simulink library "mylib"  (R2020a)
settings: Solver=VariableStepAuto  StartTime=0.0  StopTime=10.0  RelTol=1e-3
undefined symbols (not defined in the file): d_du_max_pu, dir_to_bus1, dir_to_bus_0L, dir_to_bus_2, dir_to_line1, dir_to_line_0L, dir_to_line_2, du_max_pu, du_ph_max_pu, Fi_0, Fi_T_H, Fi_T_L, Fi_T_M, I0_calc_0L, I0_comp_H, I0_comp_L, I0_comp_M, I0_max_0L, I2_max_2, I_diff1, I_diff2, I_diff3, I_diff4, I_diff5, I_diff_to, I_hight_CT1_G, I_hight_CT2_G, I_low_CT1, I_low_CT2, I_max1, I_max2, I_max3, I_max4, I_max5, I_min_sec_CT1, I_min_sec_CT2, I_unb, Iph_max_0L, Iph_max_2, jmp_in_zone, jmp_in_zone_0L, jmp_in_zone_2, K_dop, max_min1, only_K1_0L, only_K1_2, only_K2_0L, only_K2_2, only_K3_0L, only_K3_2, P_ctl_0, PQ_Fi_ctl_0, Q_ctl_0, S_set_0, set, set1, T_fast, T_I_ctl, T_off, T_on ... (+15)
libraries: $bdroot x184, powerlib_meascontrol x97
(part 14 of 14)

== system mylib/278_dzt_v1/diff_brake/calc_brake_Ic/cut_brake_4/z_ch ==
  in1 : Inport
  in2 : Inport  Port=2
  1 : RelationalOperator  Operator===  OutDataTypeStr=boolean  RndMeth=Simplest
  2 : RelationalOperator  Operator===  OutDataTypeStr=boolean  RndMeth=Simplest
  3 : Logic  AllPortsSameDT=off  OutDataTypeStr=boolean
  36 : Constant  Value=0
  out : Outport
  wires:
  3/1 -> out/1
  2/1 -> 3/2
  1/1 -> 3/1
  36/1 -> 2/2, 1/2
  in2/1 -> 2/1
  in1/1 -> 1/1

== system mylib/278_dzt_v1/diff_brake/calc_brake_Ic/cut_brake_4/z_ch1 ==
  in1 : Inport
  in2 : Inport  Port=2
  1 : RelationalOperator  Operator===  OutDataTypeStr=boolean  RndMeth=Simplest
  2 : RelationalOperator  Operator===  OutDataTypeStr=boolean  RndMeth=Simplest
  3 : Logic  AllPortsSameDT=off  OutDataTypeStr=boolean
  36 : Constant  Value=0
  out : Outport
  wires:
  3/1 -> out/1
  2/1 -> 3/2
  1/1 -> 3/1
  36/1 -> 2/2, 1/2
  in2/1 -> 2/1
  in1/1 -> 1/1

== system mylib/278_dzt_v1/diff_brake/calc_brake_Ic/cut_brake_4/z_ch2 ==
  in1 : Inport
  in2 : Inport  Port=2
  1 : RelationalOperator  Operator===  OutDataTypeStr=boolean  RndMeth=Simplest
  2 : RelationalOperator  Operator===  OutDataTypeStr=boolean  RndMeth=Simplest
  3 : Logic  AllPortsSameDT=off  OutDataTypeStr=boolean
  36 : Constant  Value=0
  out : Outport
  wires:
  3/1 -> out/1
  2/1 -> 3/2
  1/1 -> 3/1
  36/1 -> 2/2, 1/2
  in2/1 -> 2/1
  in1/1 -> 1/1

== system mylib/st_inverse/Inverse time-delay/ANSI Inverse time-delay/Equation ANSI/Zero_check ==
  in : Inport
  Constant : Constant  Value=0
  Constant1 : Constant  Value=0.000001
  Relational Operator : RelationalOperator  Operator===  OutDataTypeStr=boolean  RndMeth=Simplest
  Switch : Switch  Criteria=u2 > Threshold
  out : Outport
  wires:
  in/1 -> Switch/3, Relational Operator/1
  Constant/1 -> Relational Operator/2
  Relational Operator/1 -> Switch/2
  Constant1/1 -> Switch/1
  Switch/1 -> out/1

== system mylib/st_inverse/Inverse time-delay/ANSI Inverse time-delay/Equation ANSI/Zero_check1 ==
  in : Inport
  Constant : Constant  Value=0
  Constant1 : Constant  Value=0.000001
  Relational Operator : RelationalOperator  Operator===  OutDataTypeStr=boolean  RndMeth=Simplest
  Switch : Switch  Criteria=u2 > Threshold
  out : Outport
  wires:
  in/1 -> Switch/3, Relational Operator/1
  Constant/1 -> Relational Operator/2
  Relational Operator/1 -> Switch/2
  Constant1/1 -> Switch/1
  Switch/1 -> out/1

== system mylib/st_inverse/Inverse time-delay/ANSI Inverse time-delay inductive disk relay/Equation ANSI_idr/Zero_check ==
  in : Inport
  Constant : Constant  Value=0
  Constant1 : Constant  Value=0.000001
  Relational Operator : RelationalOperator  Operator===  OutDataTypeStr=boolean  RndMeth=Simplest
  Switch : Switch  Criteria=u2 > Threshold
  out : Outport
  wires:
  in/1 -> Switch/3, Relational Operator/1
  Constant/1 -> Relational Operator/2
  Relational Operator/1 -> Switch/2
  Constant1/1 -> Switch/1
  Switch/1 -> out/1

== system mylib/st_inverse/Inverse time-delay/ANSI Inverse time-delay inductive disk relay/Equation ANSI_idr/Zero_check1 ==
  in : Inport
  Constant : Constant  Value=0
  Constant1 : Constant  Value=0.000001
  Relational Operator : RelationalOperator  Operator===  OutDataTypeStr=boolean  RndMeth=Simplest
  Switch : Switch  Criteria=u2 > Threshold
  out : Outport
  wires:
  in/1 -> Switch/3, Relational Operator/1
  Constant/1 -> Relational Operator/2
  Relational Operator/1 -> Switch/2
  Constant1/1 -> Switch/1
  Switch/1 -> out/1

== system mylib/st_inverse/Inverse time-delay/IEC Inverse time-delay/Equation IEC/Zero_check ==
  in : Inport
  Constant : Constant  Value=0
  Constant1 : Constant  Value=0.000001
  Relational Operator : RelationalOperator  Operator===  OutDataTypeStr=boolean  RndMeth=Simplest
  Switch : Switch  Criteria=u2 > Threshold
  out : Outport
  wires:
  in/1 -> Switch/3, Relational Operator/1
  Constant/1 -> Relational Operator/2
  Relational Operator/1 -> Switch/2
  Constant1/1 -> Switch/1
  Switch/1 -> out/1

== system mylib/st_inverse/Inverse time-delay/IEC Inverse time-delay/Equation IEC/Zero_check1 ==
  in : Inport
  Constant : Constant  Value=0
  Constant1 : Constant  Value=0.000001
  Relational Operator : RelationalOperator  Operator===  OutDataTypeStr=boolean  RndMeth=Simplest
  Switch : Switch  Criteria=u2 > Threshold
  out : Outport
  wires:
  in/1 -> Switch/3, Relational Operator/1
  Constant/1 -> Relational Operator/2
  Relational Operator/1 -> Switch/2
  Constant1/1 -> Switch/1
  Switch/1 -> out/1

== system mylib/st_inverse/Inverse time-delay/IEC Inverse time-delay inductive disk relay/Equation IEC_idr/Zero_check ==
  in : Inport
  Constant : Constant  Value=0
  Constant1 : Constant  Value=0.000001
  Relational Operator : RelationalOperator  Operator===  OutDataTypeStr=boolean  RndMeth=Simplest
  Switch : Switch  Criteria=u2 > Threshold
  out : Outport
  wires:
  in/1 -> Switch/3, Relational Operator/1
  Constant/1 -> Relational Operator/2
  Relational Operator/1 -> Switch/2
  Constant1/1 -> Switch/1
  Switch/1 -> out/1

== system mylib/st_inverse/Inverse time-delay/IEC Inverse time-delay inductive disk relay/Equation IEC_idr/Zero_check1 ==
  in : Inport
  Constant : Constant  Value=0
  Constant1 : Constant  Value=0.000001
  Relational Operator : RelationalOperator  Operator===  OutDataTypeStr=boolean  RndMeth=Simplest
  Switch : Switch  Criteria=u2 > Threshold
  out : Outport
  wires:
  in/1 -> Switch/3, Relational Operator/1
  Constant/1 -> Relational Operator/2
  Relational Operator/1 -> Switch/2
  Constant1/1 -> Switch/1
  Switch/1 -> out/1
